simulink model "maglev_bearing_platform"  (R2025a)
settings: Solver=ode4  StartTime=0.0  StopTime=5  FixedStep=1e-5  RelTol=1e-3  AbsTol=1e-3  EnableMultiTasking=on
InitFcn:
  | clear;
  | H = 0.035;
  | platform_radius = 0.1;
  | floater_hight = 0.03;
  | floater_radius = 0.01;
  | 
  | air_gap = 5.1e-4;
  | k_0 = 5.4414e-07;
  | 
  | Rz = @(th) [cos(th), -sin(th), 0; sin(th), cos(th), 0; 0, 0, 1];
  | Ry = @(th) [cos(th), 0, sin(th); 0, 1, 0; -sin(th), 0, cos(th)];
  | Rx = @(th) [1, 0, 0; 0, cos(th), -sin(th); 0, sin(th), cos(th)];
  | 
  | cross_matrix = @(a) [0, -a(3), a(2); a(3), 0, -a(1); -a(2), a(1), 0];
  | 
  | %% frame-platform to frame-mb0
  | R0 = Ry(deg2rad(-90)) * Rz(deg2rad(-90));
  | t0 = [(floater_hight * 0.5 + platform_radius); 0; -H];
  | 
  | T_mb0_2_platform = [R0, t0; 0, 0, 0, 1];
  | 
  | %% frame-platform to frame-mb1
  | R1 = Rz(deg2rad(-60)) * Ry(deg2rad(90)) * Rz(deg2rad(90));
  | t1 = [(floater_hight * 0.5 + platform_radius) * cos(pi/3*2); ...
  | (floater_hight * 0.5 + platform_radius) * sin(pi/3*2); -H];
  | 
  | T_mb1_2_platform = [R1, t1; 0, 0, 0, 1];
  | 
  | %% frame-platform to frame-mb2
  | 
  | R2 = Rz(deg2rad(60)) * Ry(deg2rad(90)) * Rz(deg2rad(90));
  | t2 = [(floater_hight * 0.5 + platform_radius) * cos(pi/3*4); ...
  | (floater_hight * 0.5 + platform_radius) * sin(pi/3*4); -H];
  | 
  | T_mb2_2_platform = [R2, t2; 0, 0, 0, 1];
  | 
  | %% mb0_fx, mb0_fy -> fx, fy, fz, tx, ty, tz
  | 
  | r0_fp = T_mb0_2_platform * [0 0 0 1]';
  | 
  | F0 = R0(:, 1:2);
  | 
  | T0 = cross_matrix(r0_fp) * R0;
  | T0 = T0(:, 1:2);
  | 
  | FT0 = [F0; T0];
  | 
  | %% mb1_fx, mb1_fy -> fx, fy, fz, tx, ty, tz
  | 
  | r1_fp = T_mb1_2_platform * [0 0 0 1]';
  | 
  | F1 = R1(:, 1:2);
  | 
  | T1 = cross_matrix(r1_fp) * R1;
  | T1 = T1(:, 1:2);
  | 
  | FT1 = [F1; T1];
  | 
  | %% mb2_fx, mb1_fy -> fx, fy, fz, tx, ty, tz
  | 
  | ... (+11 lines)
undefined symbols (not defined in the file or in its folder): X, Y, Z
libraries: sm_lib x35, nesl_utility x17, simulink x1
(part 3 of 3)

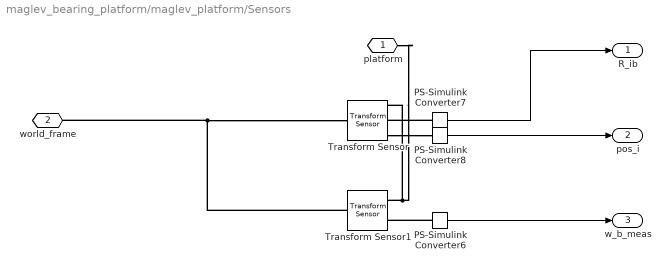
== system maglev_bearing_platform/maglev_platform/Sensors ==
  PS-Simulink Converter6 : nesl_utility/PS-Simulink Converter  PhysicalDomain=network_engine_domain  SubClassName=ps_output  LeftPortType=input  RightPortType=output  PseudoPeriodic=off  Frequencies=[]  VectorFormat=inherit  Unit=inherit  AffineConversion=off
  PS-Simulink Converter7 : nesl_utility/PS-Simulink Converter  PhysicalDomain=network_engine_domain  SubClassName=ps_output  LeftPortType=input  RightPortType=output  PseudoPeriodic=off  Frequencies=[]  VectorFormat=inherit  Unit=inherit  AffineConversion=off
  PS-Simulink Converter8 : nesl_utility/PS-Simulink Converter  PhysicalDomain=network_engine_domain  SubClassName=ps_output  LeftPortType=input  RightPortType=output  PseudoPeriodic=off  Frequencies=[]  VectorFormat=inherit  Unit=inherit  AffineConversion=off
  Transform Sensor : sm_lib/Frames and Transforms/Transform Sensor  MeasurementFrame=World  RotationSequence=ZYX  SenseAngle=off  SenseAxis=off  SenseQ=off  SenseR=on  SenseRotationSequence=off  SenseOmegaX=off  SenseOmegaY=off  SenseOmegaZ=off  SenseOmega=off  SenseQDot=off  SenseRDot=off  SenseRotationSequenceDot=off  SenseAlphaX=off  SenseAlphaY=off  SenseAlphaZ=off  SenseAlpha=off  SenseQDDot=off  SenseRDDot=off  SenseX=off  SenseY=off  SenseZ=off  SenseXYZ=on  SenseRad=off  SenseAzim=off  SenseDist=off  SenseInc=off  SenseXDot=off  SenseYDot=off  SenseZDot=off  SenseXYZDot=off  SenseRadDot=off  SenseAzimDot=off  SenseDistDot=off  SenseIncDot=off  SenseXDDot=off  SenseYDDot=off  SenseZDDot=off  SenseXYZDDot=off  SenseRadDDot=off  SenseAzimDDot=off  SenseDistDDot=off  SenseIncDDot=off
  Transform Sensor1 : sm_lib/Frames and Transforms/Transform Sensor  MeasurementFrame=Follower  RotationSequence=ZYX  SenseAngle=off  SenseAxis=off  SenseQ=off  SenseR=off  SenseRotationSequence=off  SenseOmegaX=off  SenseOmegaY=off  SenseOmegaZ=off  SenseOmega=on  SenseQDot=off  SenseRDot=off  SenseRotationSequenceDot=off  SenseAlphaX=off  SenseAlphaY=off  SenseAlphaZ=off  SenseAlpha=off  SenseQDDot=off  SenseRDDot=off  SenseX=off  SenseY=off  SenseZ=off  SenseXYZ=off  SenseRad=off  SenseAzim=off  SenseDist=off  SenseInc=off  SenseXDot=off  SenseYDot=off  SenseZDot=off  SenseXYZDot=off  SenseRadDot=off  SenseAzimDot=off  SenseDistDot=off  SenseIncDot=off  SenseXDDot=off  SenseYDDot=off  SenseZDDot=off  SenseXYZDDot=off  SenseRadDDot=off  SenseAzimDDot=off  SenseDistDDot=off  SenseIncDDot=off
  platform : PMIOPort  Side=Left
  world_frame : PMIOPort  Port=2  Side=Left
  R_ib : Outport
  pos_i : Outport  Port=2
  w_b_meas : Outport  Port=3
  wires:
  PS-Simulink Converter7/1 -> R_ib/1
  PS-Simulink Converter8/1 -> pos_i/1
  PS-Simulink Converter6/1 -> w_b_meas/1
  connections:
  Transform Sensor/RConn3 -- PS-Simulink Converter8/LConn1
  PS-Simulink Converter6/LConn1 -- Transform Sensor1/RConn2
  Transform Sensor1/RConn1 -- platform/RConn1 -- Transform Sensor/RConn1
  PS-Simulink Converter7/LConn1 -- Transform Sensor/RConn2
  Transform Sensor1/LConn1 -- world_frame/RConn1 -- Transform Sensor/LConn1

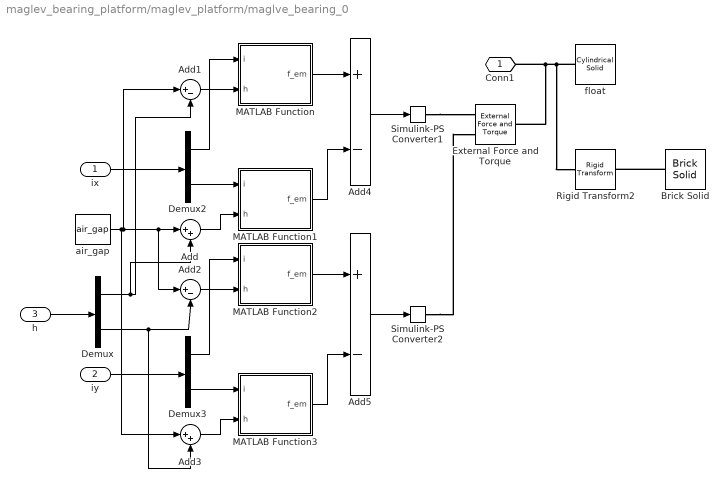
== system maglev_bearing_platform/maglev_platform/maglve_bearing_0 ==
  ix : Inport
  iy : Inport  Port=2
  h : Inport  Port=3
  Add : Sum  Inputs=|++
  Add1 : Sum  Inputs=|+-
  Add2 : Sum  Inputs=|+-
  Add3 : Sum  Inputs=|++
  Add4 : Sum  Inputs=+-
  Add5 : Sum  Inputs=+-
  Brick Solid : sm_lib/Body Elements/Brick Solid  BrickDimensions=[floater_radius*2 floater_radius*2 H+floater_radius]  BrickDimensionsUnits=m  ExportEntireGeometry=off  InertiaType=CalculateFromGeometry  BasedOnType=Density  Density=1000  DensityUnits=kg/m^3  Mass=1  MassUnits=kg  CenterOfMass=[0 0 0]  CenterOfMassUnits=m  MomentsOfInertia=[1 1 1]  MomentsOfInertiaUnits=kg*m^2  ProductsOfInertia=[0 0 0]  ProductsOfInertiaUnits=kg*m^2  GraphicType=FromGeometry  MarkerShape=Sphere  MarkerSize=10  GraphicVisPropType=SimpleVisualProperties  GraphicDiffuseColor=[1 0.6667 1]  GraphicOpacity=1  GraphicSpecularColor=[0.5 0.5 0.5 1.0]  GraphicAmbientColor=[0.15 0.15 0.15 1.0]  GraphicEmissiveColor=[0.0 0.0 0.0 1.0]  GraphicShininess=75  DoExposeReferenceFrame=on  SerializedFrames=<Frames/>
  Demux : Demux  Outputs=2
  Demux2 : Demux  Outputs=2
  Demux3 : Demux  Outputs=2
  External Force and Torque : sm_lib/Forces and Torques/External Force and Torque  EnableForceX=on  EnableForceY=on  EnableForceZ=off  EnableForce=off  ForceResolutionFrame=AttachedFrame  EnableTorqueX=off  EnableTorqueY=off  EnableTorqueZ=off  EnableTorque=off  TorqueResolutionFrame=AttachedFrame
  MATLAB Function : MATLAB Function  TreatAsAtomicUnit=on
  MATLAB Function1 : MATLAB Function  TreatAsAtomicUnit=on
  MATLAB Function2 : MATLAB Function  TreatAsAtomicUnit=on
  MATLAB Function3 : MATLAB Function  TreatAsAtomicUnit=on
  Rigid Transform2 : sm_lib/Frames and Transforms/Rigid Transform  RotationMethod=RotationSequence  FollAlignAxisA=+Z  BaseAlignAxisA=+Y  FollAlignAxisB=+Y  BaseAlignAxisB=+Z  RotationStandardAxis=+X  RotationAngle=90  RotationAngleUnits=deg  RotationArbitraryAxis=[0 0 1]  RotationSequenceAxes=FollowerAxes  RotationSequence=YXY  RotationSequenceAngles=[0 -90 0]  RotationSequenceAnglesUnits=deg  RotationMatrix=[1 0 0;0 1 0;0 0 1]  Quaternion=[1 0 0 0]  TranslationMethod=Cartesian  TranslationCartesianOffset=[0 H/2-floater_radius/2 floater_hight/2+floater_radius]  TranslationCartesianOffsetUnits=m  TranslationStandardAxis=+Y  TranslationStandardOffset=-0.0866  TranslationStandardOffsetUnits=m  TranslationROffset=0  TranslationROffsetUnits=m  TranslationThetaOffset=0  TranslationThetaOffsetUnits=deg  TranslationZOffset=0  TranslationZOffsetUnits=m
  Simulink-PS Converter1 : nesl_utility/Simulink-PS Converter  PhysicalDomain=network_engine_domain  SubClassName=ps_input  LeftPortType=input  RightPortType=output  PseudoPeriodic=off  Frequencies=[]  NoiseDistribution=none  NoiseParameters=[]  Unit=1  AffineConversion=off  FilteringAndDerivatives=provide  SimscapeFilterOrder=1  InputFilterTimeConstant=0.001  UdotUserProvided=0
  Simulink-PS Converter2 : nesl_utility/Simulink-PS Converter  PhysicalDomain=network_engine_domain  SubClassName=ps_input  LeftPortType=input  RightPortType=output  PseudoPeriodic=off  Frequencies=[]  NoiseDistribution=none  NoiseParameters=[]  Unit=1  AffineConversion=off  FilteringAndDerivatives=provide  SimscapeFilterOrder=1  InputFilterTimeConstant=0.001  UdotUserProvided=0
  air_gap : Constant  Value=air_gap
  float : sm_lib/Body Elements/Cylindrical Solid  CylinderRadius=floater_radius  CylinderRadiusUnits=m  CylinderLength=floater_hight  CylinderLengthUnits=m  ExportEntireGeometry=off  InertiaType=CalculateFromGeometry  BasedOnType=Density  Density=1000  DensityUnits=kg/m^3  Mass=1  MassUnits=kg  CenterOfMass=[0 0 0]  CenterOfMassUnits=m  MomentsOfInertia=[1 1 1]  MomentsOfInertiaUnits=kg*m^2  ProductsOfInertia=[0 0 0]  ProductsOfInertiaUnits=kg*m^2  GraphicType=FromGeometry  MarkerShape=Sphere  MarkerSize=10  GraphicVisPropType=SimpleVisualProperties  GraphicDiffuseColor=[1 0.6667 1]  GraphicOpacity=1  GraphicSpecularColor=[0.5 0.5 0.5 1.0]  GraphicAmbientColor=[0.15 0.15 0.15 1.0]  GraphicEmissiveColor=[0.0 0.0 0.0 1.0]  GraphicShininess=75  DoExposeReferenceFrame=on  SerializedFrames=<Frames/>
  Conn1 : PMIOPort  Side=Left
  wires:
  Add3/1 -> MATLAB Function3/2(h)
  Demux2/1 -> MATLAB Function/1(i)
  h/1 -> Demux/1
  MATLAB Function2/1(f_em) -> Add5/1
  air_gap/1 -> Add2/1, Add/1, Add1/1, Add3/1
  Demux/1 -> Add1/2, Add/2
  Demux/2 -> Add3/2, Add2/2
  Add1/1 -> MATLAB Function/2(h)
  Demux2/2 -> MATLAB Function1/1(i)
  Demux3/2 -> MATLAB Function3/1(i)
  Add/1 -> MATLAB Function1/2(h)
  Add2/1 -> MATLAB Function2/2(h)
  Demux3/1 -> MATLAB Function2/1(i)
  MATLAB Function/1(f_em) -> Add4/1
  MATLAB Function1/1(f_em) -> Add4/2
  MATLAB Function3/1(f_em) -> Add5/2
  Add5/1 -> Simulink-PS Converter2/1
  Add4/1 -> Simulink-PS Converter1/1
  iy/1 -> Demux3/1
  ix/1 -> Demux2/1
  connections:
  Simulink-PS Converter1/RConn1 -- External Force and Torque/LConn1
  Simulink-PS Converter2/RConn1 -- External Force and Torque/LConn2
  float/RConn1 -- Rigid Transform2/LConn1 -- Conn1/RConn1 -- External Force and Torque/RConn1
  Brick Solid/RConn1 -- Rigid Transform2/RConn1

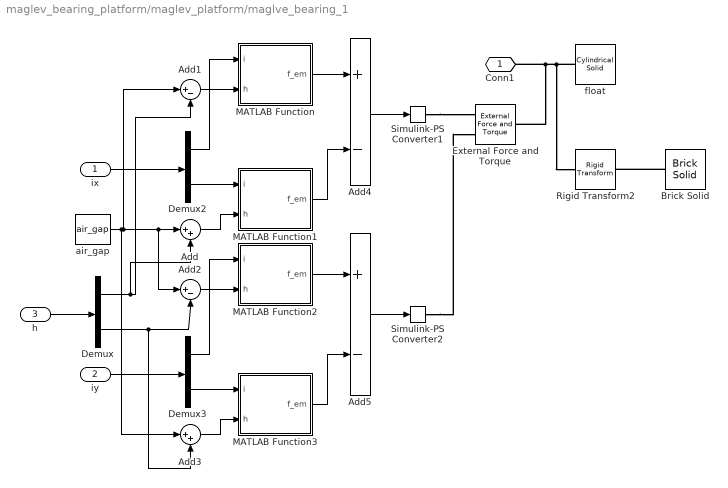
== system maglev_bearing_platform/maglev_platform/maglve_bearing_1 ==
  ix : Inport
  iy : Inport  Port=2
  h : Inport  Port=3
  Add : Sum  Inputs=|++
  Add1 : Sum  Inputs=|+-
  Add2 : Sum  Inputs=|+-
  Add3 : Sum  Inputs=|++
  Add4 : Sum  Inputs=+-
  Add5 : Sum  Inputs=+-
  Brick Solid : sm_lib/Body Elements/Brick Solid  BrickDimensions=[floater_radius*2 floater_radius*2 H+floater_radius]  BrickDimensionsUnits=m  ExportEntireGeometry=off  InertiaType=CalculateFromGeometry  BasedOnType=Density  Density=1000  DensityUnits=kg/m^3  Mass=1  MassUnits=kg  CenterOfMass=[0 0 0]  CenterOfMassUnits=m  MomentsOfInertia=[1 1 1]  MomentsOfInertiaUnits=kg*m^2  ProductsOfInertia=[0 0 0]  ProductsOfInertiaUnits=kg*m^2  GraphicType=FromGeometry  MarkerShape=Sphere  MarkerSize=10  GraphicVisPropType=SimpleVisualProperties  GraphicDiffuseColor=[1 0.6667 1]  GraphicOpacity=1  GraphicSpecularColor=[0.5 0.5 0.5 1.0]  GraphicAmbientColor=[0.15 0.15 0.15 1.0]  GraphicEmissiveColor=[0.0 0.0 0.0 1.0]  GraphicShininess=75  DoExposeReferenceFrame=on  SerializedFrames=<Frames/>
  Demux : Demux  Outputs=2
  Demux2 : Demux  Outputs=2
  Demux3 : Demux  Outputs=2
  External Force and Torque : sm_lib/Forces and Torques/External Force and Torque  EnableForceX=on  EnableForceY=on  EnableForceZ=off  EnableForce=off  ForceResolutionFrame=AttachedFrame  EnableTorqueX=off  EnableTorqueY=off  EnableTorqueZ=off  EnableTorque=off  TorqueResolutionFrame=AttachedFrame
  MATLAB Function : MATLAB Function  TreatAsAtomicUnit=on
  MATLAB Function1 : MATLAB Function  TreatAsAtomicUnit=on
  MATLAB Function2 : MATLAB Function  TreatAsAtomicUnit=on
  MATLAB Function3 : MATLAB Function  TreatAsAtomicUnit=on
  Rigid Transform2 : sm_lib/Frames and Transforms/Rigid Transform  RotationMethod=RotationSequence  FollAlignAxisA=+Z  BaseAlignAxisA=+Y  FollAlignAxisB=+Y  BaseAlignAxisB=+Z  RotationStandardAxis=+X  RotationAngle=90  RotationAngleUnits=deg  RotationArbitraryAxis=[0 0 1]  RotationSequenceAxes=FollowerAxes  RotationSequence=YXY  RotationSequenceAngles=[0 -90 0]  RotationSequenceAnglesUnits=deg  RotationMatrix=[1 0 0;0 1 0;0 0 1]  Quaternion=[1 0 0 0]  TranslationMethod=Cartesian  TranslationCartesianOffset=[0 H/2-floater_radius/2 floater_hight/2+floater_radius]  TranslationCartesianOffsetUnits=m  TranslationStandardAxis=+Y  TranslationStandardOffset=-0.0866  TranslationStandardOffsetUnits=m  TranslationROffset=0  TranslationROffsetUnits=m  TranslationThetaOffset=0  TranslationThetaOffsetUnits=deg  TranslationZOffset=0  TranslationZOffsetUnits=m
  Simulink-PS Converter1 : nesl_utility/Simulink-PS Converter  PhysicalDomain=network_engine_domain  SubClassName=ps_input  LeftPortType=input  RightPortType=output  PseudoPeriodic=off  Frequencies=[]  NoiseDistribution=none  NoiseParameters=[]  Unit=1  AffineConversion=off  FilteringAndDerivatives=provide  SimscapeFilterOrder=1  InputFilterTimeConstant=0.001  UdotUserProvided=0
  Simulink-PS Converter2 : nesl_utility/Simulink-PS Converter  PhysicalDomain=network_engine_domain  SubClassName=ps_input  LeftPortType=input  RightPortType=output  PseudoPeriodic=off  Frequencies=[]  NoiseDistribution=none  NoiseParameters=[]  Unit=1  AffineConversion=off  FilteringAndDerivatives=provide  SimscapeFilterOrder=1  InputFilterTimeConstant=0.001  UdotUserProvided=0
  air_gap : Constant  Value=air_gap
  float : sm_lib/Body Elements/Cylindrical Solid  CylinderRadius=floater_radius  CylinderRadiusUnits=m  CylinderLength=floater_hight  CylinderLengthUnits=m  ExportEntireGeometry=off  InertiaType=CalculateFromGeometry  BasedOnType=Density  Density=1000  DensityUnits=kg/m^3  Mass=1  MassUnits=kg  CenterOfMass=[0 0 0]  CenterOfMassUnits=m  MomentsOfInertia=[1 1 1]  MomentsOfInertiaUnits=kg*m^2  ProductsOfInertia=[0 0 0]  ProductsOfInertiaUnits=kg*m^2  GraphicType=FromGeometry  MarkerShape=Sphere  MarkerSize=10  GraphicVisPropType=SimpleVisualProperties  GraphicDiffuseColor=[1 0.6667 1]  GraphicOpacity=1  GraphicSpecularColor=[0.5 0.5 0.5 1.0]  GraphicAmbientColor=[0.15 0.15 0.15 1.0]  GraphicEmissiveColor=[0.0 0.0 0.0 1.0]  GraphicShininess=75  DoExposeReferenceFrame=on  SerializedFrames=<Frames/>
  Conn1 : PMIOPort  Side=Left
  wires:
  ix/1 -> Demux2/1
  iy/1 -> Demux3/1
  Add4/1 -> Simulink-PS Converter1/1
  Add5/1 -> Simulink-PS Converter2/1
  MATLAB Function3/1(f_em) -> Add5/2
  MATLAB Function1/1(f_em) -> Add4/2
  MATLAB Function/1(f_em) -> Add4/1
  Demux3/1 -> MATLAB Function2/1(i)
  Add2/1 -> MATLAB Function2/2(h)
  Add/1 -> MATLAB Function1/2(h)
  Demux3/2 -> MATLAB Function3/1(i)
  Demux2/2 -> MATLAB Function1/1(i)
  Add1/1 -> MATLAB Function/2(h)
  Demux/2 -> Add2/2, Add3/2
  Demux/1 -> Add/2, Add1/2
  air_gap/1 -> Add3/1, Add1/1, Add/1, Add2/1
  MATLAB Function2/1(f_em) -> Add5/1
  h/1 -> Demux/1
  Demux2/1 -> MATLAB Function/1(i)
  Add3/1 -> MATLAB Function3/2(h)
  connections:
  Brick Solid/RConn1 -- Rigid Transform2/RConn1
  External Force and Torque/RConn1 -- Conn1/RConn1 -- Rigid Transform2/LConn1 -- float/RConn1
  Simulink-PS Converter2/RConn1 -- External Force and Torque/LConn2
  Simulink-PS Converter1/RConn1 -- External Force and Torque/LConn1

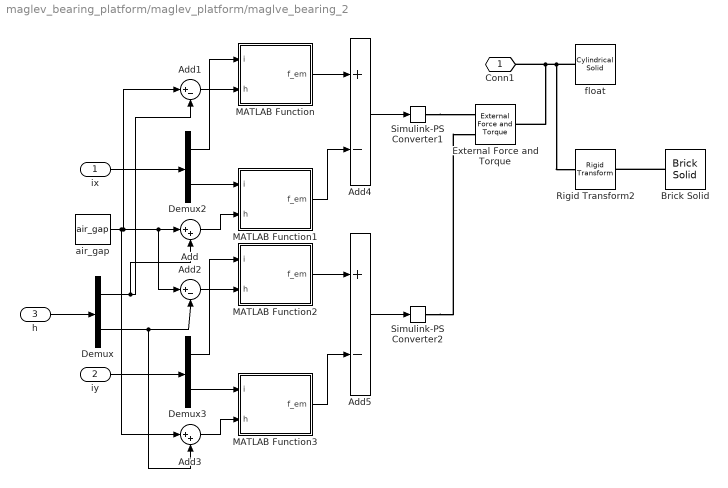
== system maglev_bearing_platform/maglev_platform/maglve_bearing_2 ==
  ix : Inport
  iy : Inport  Port=2
  h : Inport  Port=3
  Add : Sum  Inputs=|++
  Add1 : Sum  Inputs=|+-
  Add2 : Sum  Inputs=|+-
  Add3 : Sum  Inputs=|++
  Add4 : Sum  Inputs=+-
  Add5 : Sum  Inputs=+-
  Brick Solid : sm_lib/Body Elements/Brick Solid  BrickDimensions=[floater_radius*2 floater_radius*2 H+floater_radius]  BrickDimensionsUnits=m  ExportEntireGeometry=off  InertiaType=CalculateFromGeometry  BasedOnType=Density  Density=1000  DensityUnits=kg/m^3  Mass=1  MassUnits=kg  CenterOfMass=[0 0 0]  CenterOfMassUnits=m  MomentsOfInertia=[1 1 1]  MomentsOfInertiaUnits=kg*m^2  ProductsOfInertia=[0 0 0]  ProductsOfInertiaUnits=kg*m^2  GraphicType=FromGeometry  MarkerShape=Sphere  MarkerSize=10  GraphicVisPropType=SimpleVisualProperties  GraphicDiffuseColor=[1 0.6667 1]  GraphicOpacity=1  GraphicSpecularColor=[0.5 0.5 0.5 1.0]  GraphicAmbientColor=[0.15 0.15 0.15 1.0]  GraphicEmissiveColor=[0.0 0.0 0.0 1.0]  GraphicShininess=75  DoExposeReferenceFrame=on  SerializedFrames=<Frames/>
  Demux : Demux  Outputs=2
  Demux2 : Demux  Outputs=2
  Demux3 : Demux  Outputs=2
  External Force and Torque : sm_lib/Forces and Torques/External Force and Torque  EnableForceX=on  EnableForceY=on  EnableForceZ=off  EnableForce=off  ForceResolutionFrame=AttachedFrame  EnableTorqueX=off  EnableTorqueY=off  EnableTorqueZ=off  EnableTorque=off  TorqueResolutionFrame=AttachedFrame
  MATLAB Function : MATLAB Function  TreatAsAtomicUnit=on
  MATLAB Function1 : MATLAB Function  TreatAsAtomicUnit=on
  MATLAB Function2 : MATLAB Function  TreatAsAtomicUnit=on
  MATLAB Function3 : MATLAB Function  TreatAsAtomicUnit=on
  Rigid Transform2 : sm_lib/Frames and Transforms/Rigid Transform  RotationMethod=RotationSequence  FollAlignAxisA=+Z  BaseAlignAxisA=+Y  FollAlignAxisB=+Y  BaseAlignAxisB=+Z  RotationStandardAxis=+X  RotationAngle=90  RotationAngleUnits=deg  RotationArbitraryAxis=[0 0 1]  RotationSequenceAxes=FollowerAxes  RotationSequence=YXY  RotationSequenceAngles=[0 -90 0]  RotationSequenceAnglesUnits=deg  RotationMatrix=[1 0 0;0 1 0;0 0 1]  Quaternion=[1 0 0 0]  TranslationMethod=Cartesian  TranslationCartesianOffset=[0 H/2-floater_radius/2 floater_hight/2+floater_radius]  TranslationCartesianOffsetUnits=m  TranslationStandardAxis=+Y  TranslationStandardOffset=-0.0866  TranslationStandardOffsetUnits=m  TranslationROffset=0  TranslationROffsetUnits=m  TranslationThetaOffset=0  TranslationThetaOffsetUnits=deg  TranslationZOffset=0  TranslationZOffsetUnits=m
  Simulink-PS Converter1 : nesl_utility/Simulink-PS Converter  PhysicalDomain=network_engine_domain  SubClassName=ps_input  LeftPortType=input  RightPortType=output  PseudoPeriodic=off  Frequencies=[]  NoiseDistribution=none  NoiseParameters=[]  Unit=1  AffineConversion=off  FilteringAndDerivatives=provide  SimscapeFilterOrder=1  InputFilterTimeConstant=0.001  UdotUserProvided=0
  Simulink-PS Converter2 : nesl_utility/Simulink-PS Converter  PhysicalDomain=network_engine_domain  SubClassName=ps_input  LeftPortType=input  RightPortType=output  PseudoPeriodic=off  Frequencies=[]  NoiseDistribution=none  NoiseParameters=[]  Unit=1  AffineConversion=off  FilteringAndDerivatives=provide  SimscapeFilterOrder=1  InputFilterTimeConstant=0.001  UdotUserProvided=0
  air_gap : Constant  Value=air_gap
  float : sm_lib/Body Elements/Cylindrical Solid  CylinderRadius=floater_radius  CylinderRadiusUnits=m  CylinderLength=floater_hight  CylinderLengthUnits=m  ExportEntireGeometry=off  InertiaType=CalculateFromGeometry  BasedOnType=Density  Density=1000  DensityUnits=kg/m^3  Mass=1  MassUnits=kg  CenterOfMass=[0 0 0]  CenterOfMassUnits=m  MomentsOfInertia=[1 1 1]  MomentsOfInertiaUnits=kg*m^2  ProductsOfInertia=[0 0 0]  ProductsOfInertiaUnits=kg*m^2  GraphicType=FromGeometry  MarkerShape=Sphere  MarkerSize=10  GraphicVisPropType=SimpleVisualProperties  GraphicDiffuseColor=[1 0.6667 1]  GraphicOpacity=1  GraphicSpecularColor=[0.5 0.5 0.5 1.0]  GraphicAmbientColor=[0.15 0.15 0.15 1.0]  GraphicEmissiveColor=[0.0 0.0 0.0 1.0]  GraphicShininess=75  DoExposeReferenceFrame=on  SerializedFrames=<Frames/>
  Conn1 : PMIOPort  Side=Left
  wires:
  Add3/1 -> MATLAB Function3/2(h)
  Demux2/1 -> MATLAB Function/1(i)
  h/1 -> Demux/1
  MATLAB Function2/1(f_em) -> Add5/1
  air_gap/1 -> Add2/1, Add/1, Add1/1, Add3/1
  Demux/1 -> Add1/2, Add/2
  Demux/2 -> Add3/2, Add2/2
  Add1/1 -> MATLAB Function/2(h)
  Demux2/2 -> MATLAB Function1/1(i)
  Demux3/2 -> MATLAB Function3/1(i)
  Add/1 -> MATLAB Function1/2(h)
  Add2/1 -> MATLAB Function2/2(h)
  Demux3/1 -> MATLAB Function2/1(i)
  MATLAB Function/1(f_em) -> Add4/1
  MATLAB Function1/1(f_em) -> Add4/2
  MATLAB Function3/1(f_em) -> Add5/2
  Add5/1 -> Simulink-PS Converter2/1
  Add4/1 -> Simulink-PS Converter1/1
  iy/1 -> Demux3/1
  ix/1 -> Demux2/1
  connections:
  Simulink-PS Converter1/RConn1 -- External Force and Torque/LConn1
  Simulink-PS Converter2/RConn1 -- External Force and Torque/LConn2
  float/RConn1 -- Rigid Transform2/LConn1 -- Conn1/RConn1 -- External Force and Torque/RConn1
  Brick Solid/RConn1 -- Rigid Transform2/RConn1

== matlab function maglev_bearing_platform/maglev_platform/maglve_bearing_2/MATLAB Function1 ==
  data: i input; f_em output; h input; A_iron parameter; l_iron parameter; mu_0 parameter; N_coil parameter; alpha parameter; mu_iron parameter; B_sat parameter; A_a parameter
function f_em = force_em(i, h, A_iron, l_iron, mu_0, N_coil, alpha, mu_iron, B_sat, A_a)

Frolich_a = 1 / mu_iron;
Frolich_b = 1 / B_sat;
fun = @(phi) (Frolich_a * l_iron * (phi / A_iron)) / (1 - Frolich_b * abs(phi / A_iron)) ...
              + (2 * h * phi) / (mu_0 * A_a) - N_coil * i;

% 磁通上限：Phi_max = B_sat * A_iron
Phi_max = B_sat * A_iron;

Phi = fzero(fun, [0, Phi_max]);

% 麦克斯韦应力张量法计算电磁力
f_em = Phi^2 * cos(alpha) / (2 * mu_0 * A_a);

== matlab function maglev_bearing_platform/maglev_platform/maglve_bearing_2/MATLAB Function2 ==
  data: i input; f_em output; h input; A_iron parameter; l_iron parameter; mu_0 parameter; N_coil parameter; alpha parameter; mu_iron parameter; B_sat parameter; A_a parameter
function f_em = force_em(i, h, A_iron, l_iron, mu_0, N_coil, alpha, mu_iron, B_sat, A_a)

Frolich_a = 1 / mu_iron;
Frolich_b = 1 / B_sat;
fun = @(phi) (Frolich_a * l_iron * (phi / A_iron)) / (1 - Frolich_b * abs(phi / A_iron)) ...
              + (2 * h * phi) / (mu_0 * A_a) - N_coil * i;

% 磁通上限：Phi_max = B_sat * A_iron
Phi_max = B_sat * A_iron;

Phi = fzero(fun, [0, Phi_max]);

% 麦克斯韦应力张量法计算电磁力
f_em = Phi^2 * cos(alpha) / (2 * mu_0 * A_a);

== matlab function maglev_bearing_platform/maglev_platform/maglve_bearing_2/MATLAB Function3 ==
  data: i input; f_em output; h input; A_iron parameter; l_iron parameter; mu_0 parameter; N_coil parameter; alpha parameter; mu_iron parameter; B_sat parameter; A_a parameter
function f_em = force_em(i, h, A_iron, l_iron, mu_0, N_coil, alpha, mu_iron, B_sat, A_a)

Frolich_a = 1 / mu_iron;
Frolich_b = 1 / B_sat;
fun = @(phi) (Frolich_a * l_iron * (phi / A_iron)) / (1 - Frolich_b * abs(phi / A_iron)) ...
              + (2 * h * phi) / (mu_0 * A_a) - N_coil * i;

% 磁通上限：Phi_max = B_sat * A_iron
Phi_max = B_sat * A_iron;

Phi = fzero(fun, [0, Phi_max]);

% 麦克斯韦应力张量法计算电磁力
f_em = Phi^2 * cos(alpha) / (2 * mu_0 * A_a);

== matlab function maglev_bearing_platform/maglev_platform/maglve_bearing_0/MATLAB Function ==
  data: i input; f_em output; h input; A_iron parameter; l_iron parameter; mu_0 parameter; N_coil parameter; alpha parameter; mu_iron parameter; B_sat parameter; A_a parameter
function f_em = force_em(i, h, A_iron, l_iron, mu_0, N_coil, alpha, mu_iron, B_sat, A_a)

Frolich_a = 1 / mu_iron;
Frolich_b = 1 / B_sat;
fun = @(phi) (Frolich_a * l_iron * (phi / A_iron)) / (1 - Frolich_b * abs(phi / A_iron)) ...
              + (2 * h * phi) / (mu_0 * A_a) - N_coil * i;

% 磁通上限：Phi_max = B_sat * A_iron
Phi_max = B_sat * A_iron;

Phi = fzero(fun, [0, Phi_max]);

% 麦克斯韦应力张量法计算电磁力
f_em = Phi^2 * cos(alpha) / (2 * mu_0 * A_a);

== matlab function maglev_bearing_platform/maglev_platform/maglve_bearing_0/MATLAB Function1 ==
  data: i input; f_em output; h input; A_iron parameter; l_iron parameter; mu_0 parameter; N_coil parameter; alpha parameter; mu_iron parameter; B_sat parameter; A_a parameter
function f_em = force_em(i, h, A_iron, l_iron, mu_0, N_coil, alpha, mu_iron, B_sat, A_a)

Frolich_a = 1 / mu_iron;
Frolich_b = 1 / B_sat;
fun = @(phi) (Frolich_a * l_iron * (phi / A_iron)) / (1 - Frolich_b * abs(phi / A_iron)) ...
              + (2 * h * phi) / (mu_0 * A_a) - N_coil * i;

% 磁通上限：Phi_max = B_sat * A_iron
Phi_max = B_sat * A_iron;

Phi = fzero(fun, [0, Phi_max]);

% 麦克斯韦应力张量法计算电磁力
f_em = Phi^2 * cos(alpha) / (2 * mu_0 * A_a);

== matlab function maglev_bearing_platform/maglev_platform/maglve_bearing_0/MATLAB Function2 ==
  data: i input; f_em output; h input; A_iron parameter; l_iron parameter; mu_0 parameter; N_coil parameter; alpha parameter; mu_iron parameter; B_sat parameter; A_a parameter
function f_em = force_em(i, h, A_iron, l_iron, mu_0, N_coil, alpha, mu_iron, B_sat, A_a)

Frolich_a = 1 / mu_iron;
Frolich_b = 1 / B_sat;
fun = @(phi) (Frolich_a * l_iron * (phi / A_iron)) / (1 - Frolich_b * abs(phi / A_iron)) ...
              + (2 * h * phi) / (mu_0 * A_a) - N_coil * i;

% 磁通上限：Phi_max = B_sat * A_iron
Phi_max = B_sat * A_iron;

Phi = fzero(fun, [0, Phi_max]);

% 麦克斯韦应力张量法计算电磁力
f_em = Phi^2 * cos(alpha) / (2 * mu_0 * A_a);

== matlab function maglev_bearing_platform/maglev_platform/maglve_bearing_0/MATLAB Function3 ==
  data: i input; f_em output; h input; A_iron parameter; l_iron parameter; mu_0 parameter; N_coil parameter; alpha parameter; mu_iron parameter; B_sat parameter; A_a parameter
function f_em = force_em(i, h, A_iron, l_iron, mu_0, N_coil, alpha, mu_iron, B_sat, A_a)

Frolich_a = 1 / mu_iron;
Frolich_b = 1 / B_sat;
fun = @(phi) (Frolich_a * l_iron * (phi / A_iron)) / (1 - Frolich_b * abs(phi / A_iron)) ...
              + (2 * h * phi) / (mu_0 * A_a) - N_coil * i;

% 磁通上限：Phi_max = B_sat * A_iron
Phi_max = B_sat * A_iron;

Phi = fzero(fun, [0, Phi_max]);

% 麦克斯韦应力张量法计算电磁力
f_em = Phi^2 * cos(alpha) / (2 * mu_0 * A_a);

== matlab function maglev_bearing_platform/maglev_platform/maglve_bearing_1/MATLAB Function ==
  data: i input; f_em output; h input; A_iron parameter; l_iron parameter; mu_0 parameter; N_coil parameter; alpha parameter; mu_iron parameter; B_sat parameter; A_a parameter
function f_em = force_em(i, h, A_iron, l_iron, mu_0, N_coil, alpha, mu_iron, B_sat, A_a)

Frolich_a = 1 / mu_iron;
Frolich_b = 1 / B_sat;
fun = @(phi) (Frolich_a * l_iron * (phi / A_iron)) / (1 - Frolich_b * abs(phi / A_iron)) ...
              + (2 * h * phi) / (mu_0 * A_a) - N_coil * i;

% 磁通上限：Phi_max = B_sat * A_iron
Phi_max = B_sat * A_iron;

Phi = fzero(fun, [0, Phi_max]);

% 麦克斯韦应力张量法计算电磁力
f_em = Phi^2 * cos(alpha) / (2 * mu_0 * A_a);

== matlab function maglev_bearing_platform/limits/limit_mb0 ==
  data: xy input size=[2,1]; max_xy output size=[2,1]; min_xy output size=[2,1]; air_gap parameter; i_max parameter; k_0 parameter
function [max_xy, min_xy] = force_limit(xy, air_gap, i_max, k_0)
    force_x_max = k_0 * i_max * i_max / (air_gap - xy(1)) / (air_gap - xy(1));
    force_x_min = -k_0 * i_max * i_max / (air_gap + xy(1)) / (air_gap + xy(1));
    force_y_max = k_0 * i_max * i_max / (air_gap - xy(2)) / (air_gap - xy(2));
    force_y_min = -k_0 * i_max * i_max / (air_gap + xy(2)) / (air_gap + xy(2));
    max_xy = [force_x_max; force_y_max];
    min_xy = [force_x_min; force_y_min];

== matlab function maglev_bearing_platform/limits/limit_mb1 ==
  data: xy input size=[2,1]; max_xy output size=[2,1]; min_xy output size=[2,1]; air_gap parameter; i_max parameter; k_0 parameter
function [max_xy, min_xy] = force_limit(xy, air_gap, i_max, k_0)
    force_x_max = k_0 * i_max * i_max / (air_gap - xy(1)) / (air_gap - xy(1));
    force_x_min = -k_0 * i_max * i_max / (air_gap + xy(1)) / (air_gap + xy(1));
    force_y_max = k_0 * i_max * i_max / (air_gap - xy(2)) / (air_gap - xy(2));
    force_y_min = -k_0 * i_max * i_max / (air_gap + xy(2)) / (air_gap + xy(2));
    max_xy = [force_x_max; force_y_max];
    min_xy = [force_x_min; force_y_min];

== matlab function maglev_bearing_platform/limits/limit_mb2 ==
  data: xy input size=[2,1]; max_xy output size=[2,1]; min_xy output size=[2,1]; air_gap parameter; i_max parameter; k_0 parameter
function [max_xy, min_xy] = force_limit(xy, air_gap, i_max, k_0)
    force_x_max = k_0 * i_max * i_max / (air_gap - xy(1)) / (air_gap - xy(1));
    force_x_min = -k_0 * i_max * i_max / (air_gap + xy(1)) / (air_gap + xy(1));
    force_y_max = k_0 * i_max * i_max / (air_gap - xy(2)) / (air_gap - xy(2));
    force_y_min = -k_0 * i_max * i_max / (air_gap + xy(2)) / (air_gap + xy(2));
    max_xy = [force_x_max; force_y_max];
    min_xy = [force_x_min; force_y_min];

== matlab function maglev_bearing_platform/attitude_controller/MATLAB Function ==
  data: R_cmd input; tau_cmd output; R_cur input; w_b input; Kp parameter; Kd parameter
function tau_cmd = controller(R_cmd, R_cur, w_b, Kp, Kd)
    % 姿态控制器 (SO(3) 几何控制)
    % 输入：
    %   R_cmd    : 3x3 目标姿态旋转矩阵
    %   R_cur    : 3x3 当前姿态旋转矩阵
    %   w_b      : 3x1 当前角速度 (体坐标系)
    %   Kp, Kd   : 标量增益
    % 输出：
    %   tau_cmd  : 3x1 输出的命令力矩
 

    % 姿态误差（旋转向量）
    error = rotmat2vec3d(R_cur' * R_cmd);

    % PD 控制律
    tau_cmd = Kp * error' - Kd * w_b;

== matlab function maglev_bearing_platform/MATLAB Function ==
  data: u input; y output
function y = fcn(u)
theta = pi / 180 * 0.2 * sin(u);
y = [cos(theta), -sin(theta), 0; sin(theta), cos(theta), 0; 0, 0, 1];

== matlab function maglev_bearing_platform/Subsystem3/tau_2_current ==
  data: tau_cmd input; i output size=[12,1]; max_lim input; min_lim input; xy input; k_0 parameter; air_gap parameter; i_max parameter
function i = tau_2_current(tau_cmd, max_lim, min_lim, xy, k_0, air_gap, i_max)

    tau_lim = uniformScaleClip(tau_cmd, min_lim, max_lim);
    
    tau_pos = (tau_lim >= 0) .* tau_lim;
    i_1 = sqrt(tau_pos ./ k_0) .* (air_gap * ones(size(xy)) - xy);
    i_1 = min(i_1, i_max);

    tau_neg = (tau_lim < 0) .* tau_lim;
    i_2 = sqrt(-tau_neg ./ k_0) .* (air_gap * ones(size(xy)) + xy);
    i_2 = min(i_2, i_max);
    
    i_ctrl = [i_1 i_2];
    i_ctrl = i_ctrl';

    i = i_ctrl(:);

== matlab function maglev_bearing_platform/maglev_platform/maglve_bearing_1/MATLAB Function1 ==
  data: i input; f_em output; h input; A_iron parameter; l_iron parameter; mu_0 parameter; N_coil parameter; alpha parameter; mu_iron parameter; B_sat parameter; A_a parameter
function f_em = force_em(i, h, A_iron, l_iron, mu_0, N_coil, alpha, mu_iron, B_sat, A_a)

Frolich_a = 1 / mu_iron;
Frolich_b = 1 / B_sat;
fun = @(phi) (Frolich_a * l_iron * (phi / A_iron)) / (1 - Frolich_b * abs(phi / A_iron)) ...
              + (2 * h * phi) / (mu_0 * A_a) - N_coil * i;

% 磁通上限：Phi_max = B_sat * A_iron
Phi_max = B_sat * A_iron;

Phi = fzero(fun, [0, Phi_max]);

% 麦克斯韦应力张量法计算电磁力
f_em = Phi^2 * cos(alpha) / (2 * mu_0 * A_a);

== matlab function maglev_bearing_platform/maglev_platform/maglve_bearing_1/MATLAB Function2 ==
  data: i input; f_em output; h input; A_iron parameter; l_iron parameter; mu_0 parameter; N_coil parameter; alpha parameter; mu_iron parameter; B_sat parameter; A_a parameter
function f_em = force_em(i, h, A_iron, l_iron, mu_0, N_coil, alpha, mu_iron, B_sat, A_a)

Frolich_a = 1 / mu_iron;
Frolich_b = 1 / B_sat;
fun = @(phi) (Frolich_a * l_iron * (phi / A_iron)) / (1 - Frolich_b * abs(phi / A_iron)) ...
              + (2 * h * phi) / (mu_0 * A_a) - N_coil * i;

% 磁通上限：Phi_max = B_sat * A_iron
Phi_max = B_sat * A_iron;

Phi = fzero(fun, [0, Phi_max]);

% 麦克斯韦应力张量法计算电磁力
f_em = Phi^2 * cos(alpha) / (2 * mu_0 * A_a);

== matlab function maglev_bearing_platform/maglev_platform/maglve_bearing_1/MATLAB Function3 ==
  data: i input; f_em output; h input; A_iron parameter; l_iron parameter; mu_0 parameter; N_coil parameter; alpha parameter; mu_iron parameter; B_sat parameter; A_a parameter
function f_em = force_em(i, h, A_iron, l_iron, mu_0, N_coil, alpha, mu_iron, B_sat, A_a)

Frolich_a = 1 / mu_iron;
Frolich_b = 1 / B_sat;
fun = @(phi) (Frolich_a * l_iron * (phi / A_iron)) / (1 - Frolich_b * abs(phi / A_iron)) ...
              + (2 * h * phi) / (mu_0 * A_a) - N_coil * i;

% 磁通上限：Phi_max = B_sat * A_iron
Phi_max = B_sat * A_iron;

Phi = fzero(fun, [0, Phi_max]);

% 麦克斯韦应力张量法计算电磁力
f_em = Phi^2 * cos(alpha) / (2 * mu_0 * A_a);

== matlab function maglev_bearing_platform/maglev_platform/maglve_bearing_2/MATLAB Function ==
  data: i input; f_em output; h input; A_iron parameter; l_iron parameter; mu_0 parameter; N_coil parameter; alpha parameter; mu_iron parameter; B_sat parameter; A_a parameter
function f_em = force_em(i, h, A_iron, l_iron, mu_0, N_coil, alpha, mu_iron, B_sat, A_a)

Frolich_a = 1 / mu_iron;
Frolich_b = 1 / B_sat;
fun = @(phi) (Frolich_a * l_iron * (phi / A_iron)) / (1 - Frolich_b * abs(phi / A_iron)) ...
              + (2 * h * phi) / (mu_0 * A_a) - N_coil * i;

% 磁通上限：Phi_max = B_sat * A_iron
Phi_max = B_sat * A_iron;

Phi = fzero(fun, [0, Phi_max]);

% 麦克斯韦应力张量法计算电磁力
f_em = Phi^2 * cos(alpha) / (2 * mu_0 * A_a);
